simulink model "Automatic_Movement"  (R2015a)
settings: Solver=ode45  StartTime=0.0  StopTime=inf  FixedStep=0.05  RelTol=1e-3
values from neighbouring files (symbols this model uses):
  a_1 = 10.2    [Parameters.m]
  a_2 = 13.1    [Parameters.m]
  a_3 = 5.5    [Parameters.m]
  a_4 = 17    [Parameters.m]
  a_5 = 16.5    [Parameters.m]
  b_1 = 0.243    [Parameters.m]
  b_2 = 0.175    [Parameters.m]
  b_3 = 0.14    [Parameters.m]
  b_4 = 0.14    [Parameters.m]
  b_5 = 0.15    [Parameters.m]
  k1_1 = 2*alpha-a_1    (= 13.8)    [Parameters.m]
  k1_2 = 2*alpha-a_2    (= 10.9)    [Parameters.m]
  k1_3 = 2*alpha-a_3    (= 18.5)    [Parameters.m]
  k1_4 = 2*alpha-a_4    (= 7)    [Parameters.m]
  k1_5 = 2*alpha-a_5    (= 7.5)    [Parameters.m]
  k2_1 = alpha^2-b_1*k1_1    (= 140.6466)    [Parameters.m]
  k2_2 = alpha^2-b_2*k1_2    (= 142.0925)    [Parameters.m]
  k2_3 = alpha^2-b_3*k1_3    (= 141.41)    [Parameters.m]
  k2_4 = alpha^2-b_4*k1_4    (= 143.02)    [Parameters.m]
  k2_5 = alpha^2-b_5*k1_5    (= 142.875)    [Parameters.m]
  Ts = 0.06    [Parameters.m]
  Va = 24    [Parameters.m]
undefined symbols (not defined in the file or in its folder): DiscIntNeverNeededParam, gray, none, strel, videoinput
libraries: simulink x33, arduino_io_lib x28, visiontextngfix x6, visionanalysis x6, visionmorphops x4, visionstatistics x2, visionsinks x2, imaqlib x1
(part 2 of 2)

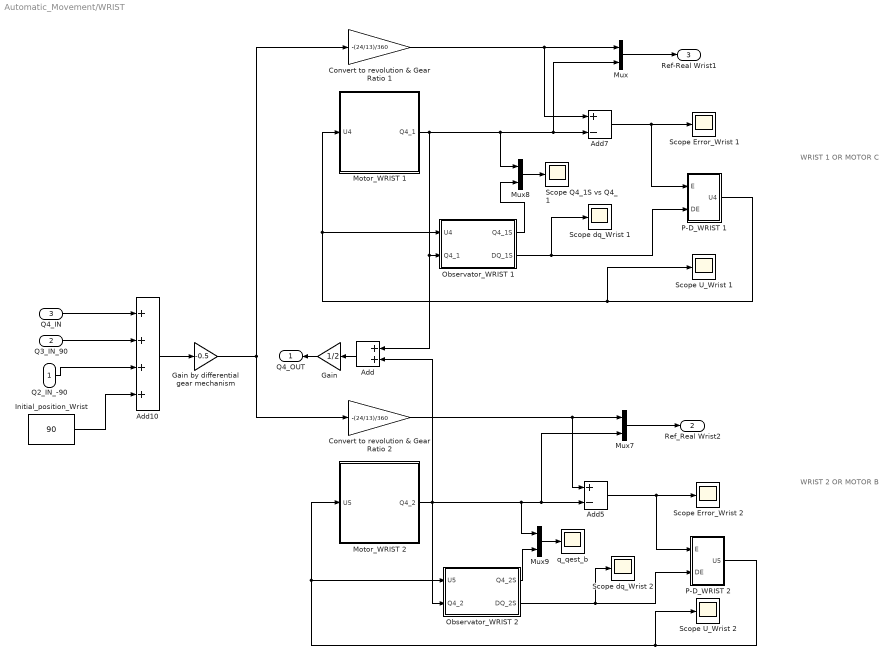
== system Automatic_Movement/WRIST ==
  note: WRIST 1
      | OR
      | MOTOR C
  note: WRIST 2
      | OR
      | MOTOR B
  Q2_IN_-90 : Inport
  "Q3_IN_90 " : Inport  Port=2
  Q4_IN : Inport  Port=3
  Add : Sum
  Add10 : Sum  Inputs=++++
  Add5 : Sum  Inputs=+-
  Add7 : Sum  Inputs=+-
  Convert to revolution & Gear Ratio 1 : Gain  Gain=-(24/13)/360
  Convert to revolution & Gear Ratio 2 : Gain  Gain=-(24/13)/360
  Gain : Gain  Gain=1/2
  Gain by differential gear mechanism : Gain  Gain=-0.5
  Initial_position_Wrist : Constant  Value=90  SampleTime=Ts
  Motor_WRIST 1 : Subsystem
  Motor_WRIST 2 : Subsystem
  Mux{,7..9} (4 alike) : Mux  Inputs=2
  Observator_WRIST 1 : Subsystem
  Observator_WRIST 2 : Subsystem
  P-D_WRIST 1 : Subsystem
  P-D_WRIST 2 : Subsystem
  Scope Error_Wrist 1 : Scope
      settings: TimeRange=auto  MaxDataPoints=5000  SaveName=e_motorc  YMin=-0.01356  YMax=0.08445  SampleTime=-1
  Scope Error_Wrist 2 : Scope
      settings: TimeRange=auto  MaxDataPoints=5000  SaveName=e_motorb  YMin=-0.00284  YMax=0.02557  SampleTime=-1
  Scope Q4_1S vs Q4_1 : Scope
      settings: TimeRange=100  MaxDataPoints=5000  SaveToWorkspace=off  SaveName=ScopeData4  YMin=-0.08445  YMax=0.01356  SampleTime=-1
  Scope U_Wrist 1 : Scope
      settings: TimeRange=auto  MaxDataPoints=5000  SaveName=u_c  YMin=-0.26048  YMax=2.34429  SampleTime=-1
  Scope U_Wrist 2 : Scope
      settings: TimeRange=auto  MaxDataPoints=5000  SaveName=u_b  YMin=-0.19737  YMax=0.74892  SampleTime=-1
  Scope dq_Wrist 1 : Scope
      settings: TimeRange=auto  MaxDataPoints=5000  SaveName=dq_c  YMin=-0.01595  YMax=0.09161  SampleTime=-1
  Scope dq_Wrist 2 : Scope
      settings: TimeRange=auto  MaxDataPoints=5000  SaveName=dq_b  YMin=-0.13693  YMax=0.06105  SampleTime=-1
  q_qest_b : Scope
      settings: TimeRange=100  MaxDataPoints=5000  SaveToWorkspace=off  SaveName=ScopeData5  YMin=-0.00142  YMax=0.01278  SampleTime=-1
  Q4_OUT : Outport
  Ref_Real Wrist2 : Outport  Port=2
  Ref-Real Wrist1 : Outport  Port=3
  wires:
  Observator_WRIST 1/2(DQ_1S) -> Scope dq_Wrist 1/1, P-D_WRIST 1/2(DE)
  P-D_WRIST 1/1(U4) -> Motor_WRIST 1/1(U4), Observator_WRIST 1/1("U4 "), Scope U_Wrist 1/1
  P-D_WRIST 2/1(U5) -> Scope U_Wrist 2/1, Motor_WRIST 2/1(U5), Observator_WRIST 2/1(U5)
  "Q3_IN_90 "/1 -> Add10/2
  Motor_WRIST 1/1(Q4_1) -> Mux/2, Add7/2, Mux8/1, Add/1, Observator_WRIST 1/2(Q4_1)
  Add10/1 -> Gain by differential gear mechanism/1
  Convert to revolution & Gear Ratio 1/1 -> Add7/1, Mux/1
  Add5/1 -> Scope Error_Wrist 2/1, P-D_WRIST 2/1(E)
  Add7/1 -> Scope Error_Wrist 1/1, P-D_WRIST 1/1(E)
  Mux/1 -> Ref-Real Wrist1/1
  Initial_position_Wrist/1 -> Add10/4
  Convert to revolution & Gear Ratio 2/1 -> Mux7/1, Add5/1
  Mux7/1 -> Ref_Real Wrist2/1
  Q4_IN/1 -> Add10/1
  Observator_WRIST 2/1(Q4_2S) -> Mux9/2
  Mux9/1 -> q_qest_b/1
  Observator_WRIST 1/1(Q4_1S) -> Mux8/2
  Motor_WRIST 2/1(Q4_2) -> Add/2, Mux7/2, Add5/2, Mux9/1, Observator_WRIST 2/2(Q4_2)
  Mux8/1 -> Scope Q4_1S vs Q4_1/1
  Gain by differential gear mechanism/1 -> Convert to revolution & Gear Ratio 2/1, Convert to revolution & Gear Ratio 1/1
  Q2_IN_-90/1 -> Add10/3
  Observator_WRIST 2/2(DQ_2S) -> Scope dq_Wrist 2/1, P-D_WRIST 2/2(DE)
  Add/1 -> Gain/1
  Gain/1 -> Q4_OUT/1

== system Automatic_Movement/BODY/Motor_BODY ==
  U1 : Inport
  Arduino Analog Write PWM : arduino_io_lib/Arduino Analog Write  arduinoVar=Temporary arduino variable: Arduino2  arduinoPin=9  T=Ts
  Arduino Digital Write  LEFT : arduino_io_lib/Arduino Digital Write  arduinoVar=Temporary arduino variable: Arduino2  arduinoPin=7  T=Ts
  Arduino Digital Write RIGHT : arduino_io_lib/Arduino Digital Write  arduinoVar=Temporary arduino variable: Arduino2  arduinoPin=6  T=Ts
  Control_Signal : Subsystem
  Encoder Read Body : arduino_io_lib/Encoder Read  arduinoVar=Temporary arduino variable: Arduino2  encNum=2  pinA=21  pinB=20  DbDl=0  T=Ts
  Gear_Ration & Pulses : Gain  Gain=1/(144*24)
  Q1 : Outport
  wires:
  Control_Signal/2(LEFT) -> Arduino Digital Write  LEFT/1
  Gear_Ration & Pulses/1 -> Q1/1
  Control_Signal/1(PWM) -> Arduino Analog Write PWM/1
  Control_Signal/3(RIGHT) -> Arduino Digital Write RIGHT/1
  Encoder Read Body/1 -> Gear_Ration & Pulses/1
  U1/1 -> Control_Signal/1(U1)

== system Automatic_Movement/BODY/Observator_BODY ==
  note: hatx
  note: dot(hatx)
  U1 : Inport
  Q1 : Inport  Port=2
  A : Gain  Gain=[0,1;0,-a_1]  Multiplication=Matrix(K*u)
  Add : Sum  Inputs=+-
  Add1 : Sum  Inputs=+++
  B : Gain  Gain=[0;b_1]  Multiplication=Matrix(K*u)
  C : Gain  Gain=[1,0]  Multiplication=Matrix(K*u)
  Demux : Demux  Outputs=2
  Integrator : Integrator
  K : Gain  Gain=[k1_1;k2_1]  Multiplication=Matrix(K*u)
  Q2_S : Outport
  DQ_S : Outport  Port=2
  wires:
  C/1 -> Add/2
  K/1 -> Add1/3
  B/1 -> Add1/2
  A/1 -> Add1/1
  Add1/1 -> Integrator/1
  Add/1 -> K/1
  Integrator/1 -> Demux/1, C/1, A/1
  Q1/1 -> Add/1
  U1/1 -> B/1
  Demux/1 -> Q2_S/1
  Demux/2 -> DQ_S/1

== system Automatic_Movement/BODY/PI-D_BODY ==
  E : Inport
  DE : Inport  Port=2
  Add : Sum  Inputs=-+
  KD : Gain  Gain=100
  KP : Gain  Gain=400
  Saturation : Saturate  UpperLimit=24  LowerLimit=-24
  U1 : Outport
  wires:
  DE/1 -> KD/1
  KP/1 -> Add/2
  KD/1 -> Add/1
  E/1 -> KP/1
  Add/1 -> Saturation/1
  Saturation/1 -> U1/1

== system Automatic_Movement/ELBOW/Motor_ELBOW ==
  U3 : Inport
  Arduino Analog Write PWM : arduino_io_lib/Arduino Analog Write  arduinoVar=Temporary arduino variable: Arduino2  arduinoPin=11  T=Ts
  Arduino Digital Write Left : arduino_io_lib/Arduino Digital Write  arduinoVar=Temporary arduino variable: Arduino2  arduinoPin=12  T=Ts
  Arduino Digital Write Right : arduino_io_lib/Arduino Digital Write  arduinoVar=Temporary arduino variable: Arduino2  arduinoPin=13  T=Ts
  Control_Signal : Subsystem
  Encoder Read Shoulder : arduino_io_lib/Encoder Read  arduinoVar=Temporary arduino variable: Arduino2  encNum=1  pinA=18  pinB=19  DbDl=0  T=Ts
  Gear_Ration & Pulses : Gain  Gain=1/(144*24)
  Q3 : Outport
  wires:
  Gear_Ration & Pulses/1 -> Q3/1
  Encoder Read Shoulder/1 -> Gear_Ration & Pulses/1
  Control_Signal/1(PWM) -> Arduino Analog Write PWM/1
  Control_Signal/3(RIGHT) -> Arduino Digital Write Right/1
  Control_Signal/2(LEFT) -> Arduino Digital Write Left/1
  U3/1 -> Control_Signal/1(U3)

== system Automatic_Movement/ELBOW/Observator_ELBOW ==
  note: hatx
  note: dot(hatx)
  U3 : Inport
  Q3 : Inport  Port=2
  A : Gain  Gain=[0,1;0,-a_3]  Multiplication=Matrix(K*u)
  Add : Sum  Inputs=+-
  Add1 : Sum  Inputs=+++
  B : Gain  Gain=[0;b_3]  Multiplication=Matrix(K*u)
  C : Gain  Gain=[1,0]  Multiplication=Matrix(K*u)
  Demux : Demux  Outputs=2
  Integrator : Integrator
  K : Gain  Gain=[k1_3;k2_3]  Multiplication=Matrix(K*u)
  Q3_S : Outport
  DQ_S : Outport  Port=2
  wires:
  C/1 -> Add/2
  K/1 -> Add1/3
  B/1 -> Add1/2
  A/1 -> Add1/1
  Add1/1 -> Integrator/1
  Add/1 -> K/1
  Integrator/1 -> A/1, Demux/1, C/1
  Q3/1 -> Add/1
  U3/1 -> B/1
  Demux/1 -> Q3_S/1
  Demux/2 -> DQ_S/1

== system Automatic_Movement/ELBOW/PI-D_ELBOW ==
  E : Inport
  DE : Inport  Port=2
  Add2 : Sum  Inputs=+-
  Add3 : Sum  Inputs=-++
  Add4 : Sum  Inputs=+-
  Discrete-Time Integrator : DiscreteIntegrator  IntegratorMethod=Integration: Trapezoidal  InitialConditionSetting=State (most efficient)  SampleTime=Ts  ICPrevOutput=DiscIntNeverNeededParam  ICPrevScaledInput=DiscIntNeverNeededParam
  KD : Gain  Gain=110
  KI : Gain  Gain=250
  KP : Gain  Gain=385
  Ka : Gain  Gain=700
  Saturation1 : Saturate  UpperLimit=24  LowerLimit=-24
  U3 : Outport
  wires:
  Add3/1 -> Add2/1, Saturation1/1
  DE/1 -> KD/1
  KP/1 -> Add3/2
  KD/1 -> Add3/1
  Add4/1 -> KI/1
  Add2/1 -> Ka/1
  Saturation1/1 -> Add2/2, U3/1
  Ka/1 -> Add4/2
  Discrete-Time Integrator/1 -> Add3/3
  KI/1 -> Discrete-Time Integrator/1
  E/1 -> Add4/1, KP/1

== system Automatic_Movement/SHOULDER /Motor_SHOULDER  ==
  U2 : Inport
  Arduino Analog Write PWM : arduino_io_lib/Arduino Analog Write  arduinoVar=Temporary arduino variable: Arduino2  arduinoPin=10  T=Ts
  Arduino Digital Write Left : arduino_io_lib/Arduino Digital Write  arduinoVar=Temporary arduino variable: Arduino2  arduinoPin=4  T=Ts
  Arduino Digital Write Right : arduino_io_lib/Arduino Digital Write  arduinoVar=Temporary arduino variable: Arduino2  arduinoPin=5  T=Ts
  Control_Signal : Subsystem
  Encoder Read Shoulder : arduino_io_lib/Encoder Read  arduinoVar=Temporary arduino variable: Arduino2  encNum=0  pinA=2  pinB=3  DbDl=0  T=Ts
  Gear_Ration & Pulses : Gain  Gain=1/(144*24)
  Q2 : Outport
  wires:
  Encoder Read Shoulder/1 -> Gear_Ration & Pulses/1
  Gear_Ration & Pulses/1 -> Q2/1
  Control_Signal/3(RIGHT) -> Arduino Digital Write Right/1
  Control_Signal/1(PWM) -> Arduino Analog Write PWM/1
  Control_Signal/2(LEFT) -> Arduino Digital Write Left/1
  U2/1 -> Control_Signal/1(U2)

== system Automatic_Movement/SHOULDER /Observator_SHOULDER ==
  note: hatx
  note: dot(hatx)
  U2 : Inport
  Q2 : Inport  Port=2
  A : Gain  Gain=[0,1;0,-a_2]  Multiplication=Matrix(K*u)
  Add : Sum  Inputs=+-
  Add1 : Sum  Inputs=+++
  B : Gain  Gain=[0;b_2]  Multiplication=Matrix(K*u)
  C : Gain  Gain=[1,0]  Multiplication=Matrix(K*u)
  Demux : Demux  Outputs=2
  Integrator : Integrator
  K : Gain  Gain=[k1_2;k2_2]  Multiplication=Matrix(K*u)
  Q2_S : Outport
  DQ_S : Outport  Port=2
  wires:
  C/1 -> Add/2
  K/1 -> Add1/3
  B/1 -> Add1/2
  A/1 -> Add1/1
  Add1/1 -> Integrator/1
  Add/1 -> K/1
  Integrator/1 -> Demux/1, C/1, A/1
  Q2/1 -> Add/1
  U2/1 -> B/1
  Demux/1 -> Q2_S/1
  Demux/2 -> DQ_S/1

== system Automatic_Movement/SHOULDER /PI-D_SHOULDER ==
  E : Inport
  DE : Inport  Port=2
  Add1 : Sum  Inputs=+-
  Add2 : Sum  Inputs=-++
  Add4 : Sum  Inputs=+-
  Discrete-Time Integrator : DiscreteIntegrator  IntegratorMethod=Integration: Trapezoidal  InitialConditionSetting=State (most efficient)  SampleTime=Ts  ICPrevOutput=DiscIntNeverNeededParam  ICPrevScaledInput=DiscIntNeverNeededParam
  KD : Gain  Gain=126
  KI : Gain  Gain=250
  KP : Gain  Gain=350
  Saturation : Saturate  UpperLimit=24  LowerLimit=-24
  ka : Gain  Gain=700
  U2 : Outport
  wires:
  KP/1 -> Add2/2
  KD/1 -> Add2/1
  DE/1 -> KD/1
  KI/1 -> Discrete-Time Integrator/1
  ka/1 -> Add4/2
  Add1/1 -> ka/1
  Discrete-Time Integrator/1 -> Add2/3
  Add2/1 -> Add1/1, Saturation/1
  Saturation/1 -> U2/1, Add1/2
  Add4/1 -> KI/1
  E/1 -> KP/1, Add4/1

== system Automatic_Movement/Selectors/Selector_phi ==
  OPENING_GRIPPER : Inport
  CLOSING_GRIPPER : Inport  Port=2
  OPEN_SENSOR : Inport  Port=3
  FORCE_SENSOR : Inport  Port=4
  KI_CAMARA_PHI : Inport  Port=5
  KI_FIXED_PHI : Inport  Port=6
  Data Store Read No WorkSpace : DataStoreRead  DataStoreName=No_WorkSpace  SampleTime=Ts
  Logical Operator : Logic  Operator=OR  Inputs=3  AllPortsSameDT=off  OutDataTypeStr=boolean
  Logical Operator1 : Logic  Operator=OR  AllPortsSameDT=off  OutDataTypeStr=boolean
  Logical Operator3 : Logic  Operator=NOT  AllPortsSameDT=off  OutDataTypeStr=boolean
  Logical Operator5 : Logic  Operator=NOT  AllPortsSameDT=off  OutDataTypeStr=boolean
  Logical Operator6 : Logic  AllPortsSameDT=off  OutDataTypeStr=boolean
  Switch1 : Switch  Threshold=1  ZeroCross=off
  Switch8 : Switch  Threshold=1  ZeroCross=off
  K_I_PHI : Outport
  wires:
  KI_CAMARA_PHI/1 -> Switch8/1, Switch1/3
  Logical Operator/1 -> Switch8/2
  Switch8/1 -> K_I_PHI/1
  CLOSING_GRIPPER/1 -> Logical Operator/1
  OPENING_GRIPPER/1 -> Logical Operator1/1
  OPEN_SENSOR/1 -> Logical Operator/2
  KI_FIXED_PHI/1 -> Switch1/1
  Switch1/1 -> Switch8/3
  FORCE_SENSOR/1 -> Logical Operator3/1, Logical Operator1/2
  Logical Operator1/1 -> Switch1/2
  Logical Operator3/1 -> Logical Operator6/2
  Logical Operator5/1 -> Logical Operator6/1
  Data Store Read No WorkSpace/1 -> Logical Operator5/1
  Logical Operator6/1 -> Logical Operator/3

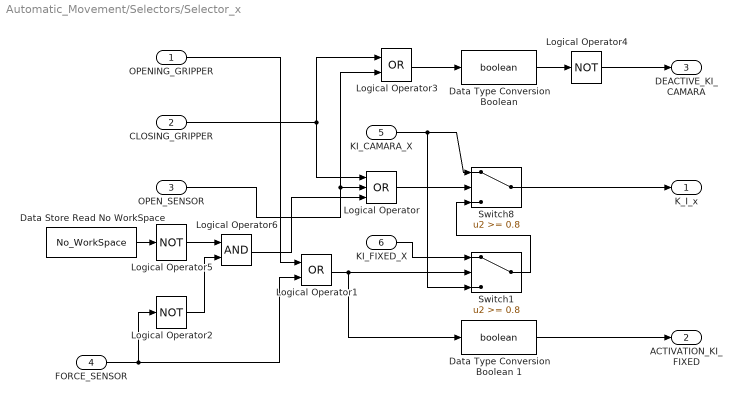
== system Automatic_Movement/Selectors/Selector_x ==
  OPENING_GRIPPER : Inport
  CLOSING_GRIPPER : Inport  Port=2
  OPEN_SENSOR : Inport  Port=3
  FORCE_SENSOR : Inport  Port=4
  KI_CAMARA_X : Inport  Port=5
  KI_FIXED_X : Inport  Port=6
  Data Store Read No WorkSpace : DataStoreRead  DataStoreName=No_WorkSpace  SampleTime=Ts
  Data Type Conversion Boolean 1 : DataTypeConversion  OutDataTypeStr=boolean
  Data Type Conversion Boolean : DataTypeConversion  OutDataTypeStr=boolean
  Logical Operator : Logic  Operator=OR  Inputs=3  AllPortsSameDT=off  OutDataTypeStr=boolean
  Logical Operator1 : Logic  Operator=OR  AllPortsSameDT=off  OutDataTypeStr=boolean
  Logical Operator2 : Logic  Operator=NOT  AllPortsSameDT=off  OutDataTypeStr=boolean
  Logical Operator3 : Logic  Operator=OR  AllPortsSameDT=off  OutDataTypeStr=boolean
  Logical Operator4 : Logic  Operator=NOT  AllPortsSameDT=off  OutDataTypeStr=boolean
  Logical Operator5 : Logic  Operator=NOT  AllPortsSameDT=off  OutDataTypeStr=boolean
  Logical Operator6 : Logic  AllPortsSameDT=off  OutDataTypeStr=boolean
  Switch1 : Switch  Threshold=0.8  ZeroCross=off
  Switch8 : Switch  Threshold=0.8  ZeroCross=off
  K_I_x : Outport
  ACTIVATION_KI_FIXED : Outport  Port=2
  DEACTIVE_KI_CAMARA : Outport  Port=3
  wires:
  KI_CAMARA_X/1 -> Switch8/1, Switch1/3
  Logical Operator/1 -> Switch8/2
  Switch8/1 -> K_I_x/1
  CLOSING_GRIPPER/1 -> Logical Operator3/1, Logical Operator/1
  OPENING_GRIPPER/1 -> Logical Operator1/1
  OPEN_SENSOR/1 -> Logical Operator/2, Logical Operator3/2
  KI_FIXED_X/1 -> Switch1/1
  Switch1/1 -> Switch8/3
  FORCE_SENSOR/1 -> Logical Operator1/2, Logical Operator2/1
  Logical Operator1/1 -> Data Type Conversion Boolean 1/1, Switch1/2
  Data Type Conversion Boolean 1/1 -> ACTIVATION_KI_FIXED/1
  Logical Operator3/1 -> Data Type Conversion Boolean/1
  Data Type Conversion Boolean/1 -> Logical Operator4/1
  Logical Operator4/1 -> DEACTIVE_KI_CAMARA/1
  Data Store Read No WorkSpace/1 -> Logical Operator5/1
  Logical Operator5/1 -> Logical Operator6/1
  Logical Operator2/1 -> Logical Operator6/2
  Logical Operator6/1 -> Logical Operator/3

== system Automatic_Movement/Selectors/Selector_y ==
  "OPENING_GRIPPER " : Inport
  CLOSING_GRIPPER : Inport  Port=2
  OPEN_SENSOR : Inport  Port=3
  FORCE_SENSOR : Inport  Port=4
  CI_CAMARA_y : Inport  Port=5
  KI_FIXED_Y : Inport  Port=6
  Data Store Read No WorkSpace : DataStoreRead  DataStoreName=No_WorkSpace  SampleTime=Ts
  Logical Operator : Logic  Operator=OR  Inputs=3  AllPortsSameDT=off  OutDataTypeStr=boolean
  Logical Operator1 : Logic  Operator=OR  AllPortsSameDT=off  OutDataTypeStr=boolean
  Logical Operator3 : Logic  Operator=NOT  AllPortsSameDT=off  OutDataTypeStr=boolean
  Logical Operator5 : Logic  Operator=NOT  AllPortsSameDT=off  OutDataTypeStr=boolean
  Logical Operator6 : Logic  AllPortsSameDT=off  OutDataTypeStr=boolean
  Switch1 : Switch  Threshold=1  ZeroCross=off
  Switch8 : Switch  Threshold=1  ZeroCross=off
  K_I_Y : Outport
  wires:
  CI_CAMARA_y/1 -> Switch1/3, Switch8/1
  Logical Operator/1 -> Switch8/2
  Switch8/1 -> K_I_Y/1
  CLOSING_GRIPPER/1 -> Logical Operator/1
  "OPENING_GRIPPER "/1 -> Logical Operator1/1
  OPEN_SENSOR/1 -> Logical Operator/2
  KI_FIXED_Y/1 -> Switch1/1
  Switch1/1 -> Switch8/3
  FORCE_SENSOR/1 -> Logical Operator3/1, Logical Operator1/2
  Logical Operator1/1 -> Switch1/2
  Data Store Read No WorkSpace/1 -> Logical Operator5/1
  Logical Operator6/1 -> Logical Operator/3
  Logical Operator3/1 -> Logical Operator6/2
  Logical Operator5/1 -> Logical Operator6/1

== system Automatic_Movement/Selectors/Selector_z ==
  OPENING_GRIPPER : Inport
  CLOSING_GRIPPER : Inport  Port=2
  OPEN_SENSOR : Inport  Port=3
  FORCE_SENSOR : Inport  Port=4
  KI_CAMARA_Z : Inport  Port=5
  KI_FIXED_Z : Inport  Port=6
  Data Store Read No WorkSpace : DataStoreRead  DataStoreName=No_WorkSpace  SampleTime=Ts
  Logical Operator : Logic  Operator=OR  Inputs=3  AllPortsSameDT=off  OutDataTypeStr=boolean
  Logical Operator1 : Logic  Operator=OR  AllPortsSameDT=off  OutDataTypeStr=boolean
  Logical Operator3 : Logic  Operator=NOT  AllPortsSameDT=off  OutDataTypeStr=boolean
  Logical Operator5 : Logic  Operator=NOT  AllPortsSameDT=off  OutDataTypeStr=boolean
  Logical Operator6 : Logic  AllPortsSameDT=off  OutDataTypeStr=boolean
  Switch1 : Switch  Threshold=1  ZeroCross=off
  Switch8 : Switch  Threshold=1  ZeroCross=off
  K_I_Z : Outport
  wires:
  KI_CAMARA_Z/1 -> Switch8/1, Switch1/3
  Logical Operator/1 -> Switch8/2
  Switch8/1 -> K_I_Z/1
  CLOSING_GRIPPER/1 -> Logical Operator/1
  OPENING_GRIPPER/1 -> Logical Operator1/1
  OPEN_SENSOR/1 -> Logical Operator/2
  KI_FIXED_Z/1 -> Switch1/1
  Switch1/1 -> Switch8/3
  FORCE_SENSOR/1 -> Logical Operator1/2, Logical Operator3/1
  Logical Operator1/1 -> Switch1/2
  Logical Operator6/1 -> Logical Operator/3
  Logical Operator3/1 -> Logical Operator6/2
  Logical Operator5/1 -> Logical Operator6/1
  Data Store Read No WorkSpace/1 -> Logical Operator5/1

== system Automatic_Movement/Vision/Enabled and Triggered Subsystem ==
  R_in : Inport
  G_in : Inport  Port=2
  B_in : Inport  Port=3
  Enable : EnablePort
  R_out : Outport
  G_out : Outport  Port=2
  B_out : Outport  Port=3
  wires:
  R_in/1 -> R_out/1
  B_in/1 -> B_out/1
  G_in/1 -> G_out/1

== system Automatic_Movement/Vision/Eval_Circle_R ==
  In1 : Inport
  Compare To Constant : simulink/Logic and Bit Operations/Compare To Constant  relop=>=  const=1.0  OutDataTypeStr=boolean
  Constant : Constant  Value=[1,1]  VectorParams1D=off
  Data Type Conversion1 : DataTypeConversion  OutDataTypeStr=double
  Dot Product : DotProduct  InputSameDT=on  OutDataTypeStr=Inherit: Inherit via internal rule
  Out1 : Outport
  wires:
  Dot Product/1 -> Compare To Constant/1
  Constant/1 -> Dot Product/1
  Data Type Conversion1/1 -> Dot Product/2
  Compare To Constant/1 -> Out1/1
  In1/1 -> Data Type Conversion1/1

== system Automatic_Movement/Vision/Eval_Circle_Y ==
  In1 : Inport
  Compare To Constant : simulink/Logic and Bit Operations/Compare To Constant  relop=>=  const=1.0  OutDataTypeStr=boolean
  Constant : Constant  Value=[1,1]  VectorParams1D=off
  Data Type Conversion1 : DataTypeConversion  OutDataTypeStr=double
  Dot Product : DotProduct  InputSameDT=on  OutDataTypeStr=Inherit: Inherit via internal rule
  Out1 : Outport
  wires:
  Dot Product/1 -> Compare To Constant/1
  Constant/1 -> Dot Product/1
  Data Type Conversion1/1 -> Dot Product/2
  Compare To Constant/1 -> Out1/1
  In1/1 -> Data Type Conversion1/1

== system Automatic_Movement/Vision/Eval_Square_R ==
  In1 : Inport
  Compare To Constant : simulink/Logic and Bit Operations/Compare To Constant  relop=>=  const=1.0  OutDataTypeStr=boolean
  Constant : Constant  Value=[1,1]  VectorParams1D=off
  Data Type Conversion1 : DataTypeConversion  OutDataTypeStr=double
  Dot Product : DotProduct  InputSameDT=on  OutDataTypeStr=Inherit: Inherit via internal rule
  Out1 : Outport
  wires:
  Compare To Constant/1 -> Out1/1
  Constant/1 -> Dot Product/1
  Data Type Conversion1/1 -> Dot Product/2
  Dot Product/1 -> Compare To Constant/1
  In1/1 -> Data Type Conversion1/1

== system Automatic_Movement/Vision/Eval_Square_Y ==
  In1 : Inport
  Compare To Constant : simulink/Logic and Bit Operations/Compare To Constant  relop=>=  const=1.0  OutDataTypeStr=boolean
  Constant : Constant  Value=[1,1]  VectorParams1D=off
  Data Type Conversion1 : DataTypeConversion  OutDataTypeStr=double
  Dot Product : DotProduct  InputSameDT=on  OutDataTypeStr=Inherit: Inherit via internal rule
  Out1 : Outport
  wires:
  Compare To Constant/1 -> Out1/1
  Constant/1 -> Dot Product/1
  Data Type Conversion1/1 -> Dot Product/2
  Dot Product/1 -> Compare To Constant/1
  In1/1 -> Data Type Conversion1/1

== system Automatic_Movement/Vision/Figure_Calculator_R ==
  note: Th_Square
  note: Th_Circle
  "C " : Inport
  Constant1 : Constant  Value=13.6
  Constant4 : Constant  Value=12.5
  Constant5 : Constant  Value=18
  Constant6 : Constant  Value=13.6
  Logical Operator : Logic  AllPortsSameDT=off  OutDataTypeStr=boolean
  Logical Operator2 : Logic  AllPortsSameDT=off  OutDataTypeStr=boolean
  Relational Operator : RelationalOperator  Operator=<=  OutDataTypeStr=boolean
  Relational Operator1 : RelationalOperator  Operator=>  OutDataTypeStr=boolean
  Relational Operator4 : RelationalOperator  Operator=<=  OutDataTypeStr=boolean
  Relational Operator5 : RelationalOperator  Operator=>  OutDataTypeStr=boolean
  Circle : Outport
  Square : Outport  Port=2
  wires:
  Relational Operator/1 -> Logical Operator/1
  Constant4/1 -> Relational Operator/1
  Relational Operator1/1 -> Logical Operator/2
  Logical Operator/1 -> Circle/1
  Constant1/1 -> Relational Operator1/1
  Logical Operator2/1 -> Square/1
  Relational Operator4/1 -> Logical Operator2/1
  Constant5/1 -> Relational Operator5/1
  Relational Operator5/1 -> Logical Operator2/2
  Constant6/1 -> Relational Operator4/1
  "C "/1 -> Relational Operator1/2, Relational Operator/2, Relational Operator4/2, Relational Operator5/2

== system Automatic_Movement/Vision/Figure_Calculator_Y ==
  note: Th_Square
  note: Th_Circle
  "C " : Inport
  Constant1 : Constant  Value=13.6
  Constant4 : Constant  Value=12.5
  Constant5 : Constant  Value=18
  Constant6 : Constant  Value=13.6
  Logical Operator : Logic  AllPortsSameDT=off  OutDataTypeStr=boolean
  Logical Operator2 : Logic  AllPortsSameDT=off  OutDataTypeStr=boolean
  Relational Operator : RelationalOperator  Operator=<=  OutDataTypeStr=boolean
  Relational Operator1 : RelationalOperator  Operator=>  OutDataTypeStr=boolean
  Relational Operator4 : RelationalOperator  Operator=<=  OutDataTypeStr=boolean
  Relational Operator5 : RelationalOperator  Operator=>  OutDataTypeStr=boolean
  Circle : Outport
  Square : Outport  Port=2
  wires:
  Relational Operator/1 -> Logical Operator/1
  Constant4/1 -> Relational Operator/1
  Relational Operator1/1 -> Logical Operator/2
  Logical Operator/1 -> Circle/1
  Constant1/1 -> Relational Operator1/1
  Logical Operator2/1 -> Square/1
  Relational Operator4/1 -> Logical Operator2/1
  Constant5/1 -> Relational Operator5/1
  Relational Operator5/1 -> Logical Operator2/2
  Constant6/1 -> Relational Operator4/1
  "C "/1 -> Relational Operator1/2, Relational Operator/2, Relational Operator4/2, Relational Operator5/2

== system Automatic_Movement/Vision/Filter_R ==
  Bw_in : Inport
  Dilation strel('diamond',2) : visionmorphops/Dilation  nhoodsrc=Specify via dialog  strel=strel('diamond',2)
  Erosion strel('diamond',1) : visionmorphops/Erosion  nhoodsrc=Specify via dialog  strel=strel('diamond',1)
  Bw_out : Outport
  wires:
  Erosion strel('diamond',1)/1 -> Dilation strel('diamond',2)/1
  Bw_in/1 -> Erosion strel('diamond',1)/1
  Dilation strel('diamond',2)/1 -> Bw_out/1

== system Automatic_Movement/Vision/Filter_Y ==
  Bw_in : Inport
  Dilation strel('diamond',2) : visionmorphops/Dilation  nhoodsrc=Specify via dialog  strel=strel('diamond',2)
  Erosion strel('diamond',1) : visionmorphops/Erosion  nhoodsrc=Specify via dialog  strel=strel('diamond',1)
  Bw_out : Outport
  wires:
  Erosion strel('diamond',1)/1 -> Dilation strel('diamond',2)/1
  Bw_in/1 -> Erosion strel('diamond',1)/1
  Dilation strel('diamond',2)/1 -> Bw_out/1

== system Automatic_Movement/Vision/Red_Identi ==
  R : Inport
  G : Inport  Port=2
  B : Inport  Port=3
  Logical Operator : Logic  Inputs=6  AllPortsSameDT=off  OutDataTypeStr=boolean
  Median Filter_Circular_[5 5]_B : visionanalysis/Median Filter  nghbood=[5 5]  outSize=Same as input port I  padType=Circular  padSrc=Specify via dialog  padVal=0  roundingMode=Floor  overflowMode=off
  Median Filter_Circular_[5 5]_G : visionanalysis/Median Filter  nghbood=[5 5]  outSize=Same as input port I  padType=Circular  padSrc=Specify via dialog  padVal=0  roundingMode=Floor  overflowMode=off
  Median Filter_Circular_[5 5]_R : visionanalysis/Median Filter  nghbood=[5 5]  outSize=Same as input port I  padType=Circular  padSrc=Specify via dialog  padVal=0  roundingMode=Floor  overflowMode=off
  Th_max_B : simulink/Logic and Bit Operations/Compare To Constant  relop=<=  const=(150)/255  OutDataTypeStr=boolean
  Th_max_G : simulink/Logic and Bit Operations/Compare To Constant  relop=<=  const=(150)/255  OutDataTypeStr=boolean
  "Th_max_R " : simulink/Logic and Bit Operations/Compare To Constant  relop=<=  const=(225+30)/255  OutDataTypeStr=boolean
  Th_min_B : simulink/Logic and Bit Operations/Compare To Constant  relop=>=  const=(0)/255  OutDataTypeStr=boolean
  Th_min_G : simulink/Logic and Bit Operations/Compare To Constant  relop=>=  const=(0)/255  OutDataTypeStr=boolean
  Th_min_R : simulink/Logic and Bit Operations/Compare To Constant  relop=>=  const=(225-40)/255  OutDataTypeStr=boolean
  BW : Outport
  wires:
  "Th_max_R "/1 -> Logical Operator/2
  Logical Operator/1 -> BW/1
  Th_min_B/1 -> Logical Operator/5
  Th_max_G/1 -> Logical Operator/4
  Th_min_R/1 -> Logical Operator/1
  Th_min_G/1 -> Logical Operator/3
  Th_max_B/1 -> Logical Operator/6
  R/1 -> Median Filter_Circular_[5 5]_R/1
  G/1 -> Median Filter_Circular_[5 5]_G/1
  B/1 -> Median Filter_Circular_[5 5]_B/1
  Median Filter_Circular_[5 5]_R/1 -> "Th_max_R "/1, Th_min_R/1
  Median Filter_Circular_[5 5]_G/1 -> Th_max_G/1, Th_min_G/1
  Median Filter_Circular_[5 5]_B/1 -> Th_max_B/1, Th_min_B/1

== system Automatic_Movement/Vision/Yellow_ide ==
  R : Inport
  G : Inport  Port=2
  B : Inport  Port=3
  Logical Operator : Logic  Inputs=6  AllPortsSameDT=off  OutDataTypeStr=boolean
  Median Filter_Circular_[5 5]_B : visionanalysis/Median Filter  nghbood=[5 5]  outSize=Same as input port I  padType=Circular  padSrc=Specify via dialog  padVal=0  roundingMode=Floor  overflowMode=off
  Median Filter_Circular_[5 5]_G : visionanalysis/Median Filter  nghbood=[5 5]  outSize=Same as input port I  padType=Circular  padSrc=Specify via dialog  padVal=0  roundingMode=Floor  overflowMode=off
  Median Filter_Circular_[5 5]_R : visionanalysis/Median Filter  nghbood=[5 5]  outSize=Same as input port I  padType=Circular  padSrc=Specify via dialog  padVal=0  roundingMode=Floor  overflowMode=off
  Th_max_B : simulink/Logic and Bit Operations/Compare To Constant  relop=<=  const=(200)/255  OutDataTypeStr=boolean
  Th_max_G : simulink/Logic and Bit Operations/Compare To Constant  relop=<=  const=(225+30)/255  OutDataTypeStr=boolean
  Th_max_R : simulink/Logic and Bit Operations/Compare To Constant  relop=<=  const=(225+30)/255  OutDataTypeStr=boolean
  Th_min_B : simulink/Logic and Bit Operations/Compare To Constant  relop=>=  const=(0)/255  OutDataTypeStr=boolean
  "Th_min_G " : simulink/Logic and Bit Operations/Compare To Constant  relop=>=  const=(200)/255  OutDataTypeStr=boolean
  "Th_min_R " : simulink/Logic and Bit Operations/Compare To Constant  relop=>=  const=(200)/255  OutDataTypeStr=boolean
  BW : Outport
  wires:
  Th_max_R/1 -> Logical Operator/2
  Logical Operator/1 -> BW/1
  Th_min_B/1 -> Logical Operator/5
  Th_max_G/1 -> Logical Operator/4
  "Th_min_R "/1 -> Logical Operator/1
  "Th_min_G "/1 -> Logical Operator/3
  Th_max_B/1 -> Logical Operator/6
  G/1 -> Median Filter_Circular_[5 5]_G/1
  R/1 -> Median Filter_Circular_[5 5]_R/1
  B/1 -> Median Filter_Circular_[5 5]_B/1
  Median Filter_Circular_[5 5]_R/1 -> "Th_min_R "/1, Th_max_R/1
  Median Filter_Circular_[5 5]_G/1 -> Th_max_G/1, "Th_min_G "/1
  Median Filter_Circular_[5 5]_B/1 -> Th_max_B/1, Th_min_B/1

== system Automatic_Movement/WRIST/Motor_WRIST 1 ==
  U4 : Inport
  Arduino Analog Write PWM : arduino_io_lib/Arduino Analog Write  arduinoVar=Temporary arduino variable: Arduino1  arduinoPin=10  T=Ts
  Arduino Digital Write Left : arduino_io_lib/Arduino Digital Write  arduinoVar=Temporary arduino variable: Arduino1  arduinoPin=4  T=Ts
  Arduino Digital Write Right : arduino_io_lib/Arduino Digital Write  arduinoVar=Temporary arduino variable: Arduino1  arduinoPin=5  T=Ts
  Control_Signal : Subsystem
  Encoder Read Wrist 1(C) : arduino_io_lib/Encoder Read  arduinoVar=Temporary arduino variable: Arduino1  encNum=1  pinA=19  pinB=18  DbDl=0  T=Ts
  Gear_Ration & Pulses : Gain  Gain=1/(72*48)
  Q4_1 : Outport
  wires:
  Control_Signal/3(RIGHT) -> Arduino Digital Write Right/1
  Control_Signal/1(PWM) -> Arduino Analog Write PWM/1
  Control_Signal/2(LEFT) -> Arduino Digital Write Left/1
  Encoder Read Wrist 1(C)/1 -> Gear_Ration & Pulses/1
  Gear_Ration & Pulses/1 -> Q4_1/1
  U4/1 -> Control_Signal/1(U1)

== system Automatic_Movement/WRIST/Motor_WRIST 2 ==
  U5 : Inport
  Arduino Analog Write PWM : arduino_io_lib/Arduino Analog Write  arduinoVar=Temporary arduino variable: Arduino1  arduinoPin=11  T=Ts
  Arduino Digital Write Left : arduino_io_lib/Arduino Digital Write  arduinoVar=Temporary arduino variable: Arduino1  arduinoPin=13  T=Ts
  Arduino Digital Write Right : arduino_io_lib/Arduino Digital Write  arduinoVar=Temporary arduino variable: Arduino1  arduinoPin=12  T=Ts
  Control_Signal : Subsystem
  Encoder Read Wrist 2 (B) : arduino_io_lib/Encoder Read  arduinoVar=Temporary arduino variable: Arduino1  encNum=0  pinA=3  pinB=2  DbDl=0  T=Ts
  Gear_Ration & Pulses : Gain  Gain=1/(72*22)
  Q4_2 : Outport
  wires:
  Encoder Read Wrist 2 (B)/1 -> Gear_Ration & Pulses/1
  Gear_Ration & Pulses/1 -> Q4_2/1
  Control_Signal/3(RIGHT) -> Arduino Digital Write Right/1
  Control_Signal/1(PWM) -> Arduino Analog Write PWM/1
  Control_Signal/2(LEFT) -> Arduino Digital Write Left/1
  U5/1 -> Control_Signal/1(U1)

== system Automatic_Movement/WRIST/Observator_WRIST 1 ==
  note: hatx
  note: dot(hatx)
  "U4 " : Inport
  Q4_1 : Inport  Port=2
  A : Gain  Gain=[0,1;0,-a_5]  Multiplication=Matrix(K*u)
  Add : Sum  Inputs=+-
  Add1 : Sum  Inputs=+++
  B : Gain  Gain=[0;b_5]  Multiplication=Matrix(K*u)
  C : Gain  Gain=[1,0]  Multiplication=Matrix(K*u)
  Demux : Demux  Outputs=2
  Integrator : Integrator
  K : Gain  Gain=[k1_5;k2_5]  Multiplication=Matrix(K*u)
  Q4_1S : Outport
  DQ_1S : Outport  Port=2
  wires:
  C/1 -> Add/2
  K/1 -> Add1/3
  B/1 -> Add1/2
  A/1 -> Add1/1
  Add1/1 -> Integrator/1
  Add/1 -> K/1
  Integrator/1 -> Demux/1, C/1, A/1
  Q4_1/1 -> Add/1
  "U4 "/1 -> B/1
  Demux/1 -> Q4_1S/1
  Demux/2 -> DQ_1S/1

== system Automatic_Movement/WRIST/Observator_WRIST 2 ==
  note: hatx
  note: dot(hatx)
  U5 : Inport
  Q4_2 : Inport  Port=2
  A : Gain  Gain=[0,1;0,-a_4]  Multiplication=Matrix(K*u)
  Add : Sum  Inputs=+-
  Add1 : Sum  Inputs=+++
  B : Gain  Gain=[0;b_4]  Multiplication=Matrix(K*u)
  C : Gain  Gain=[1,0]  Multiplication=Matrix(K*u)
  Demux : Demux  Outputs=2
  Integrator : Integrator
  K : Gain  Gain=[k1_4;k2_4]  Multiplication=Matrix(K*u)
  Q4_2S : Outport
  DQ_2S : Outport  Port=2
  wires:
  C/1 -> Add/2
  K/1 -> Add1/3
  B/1 -> Add1/2
  A/1 -> Add1/1
  Add1/1 -> Integrator/1
  Add/1 -> K/1
  Integrator/1 -> Demux/1, C/1, A/1
  Q4_2/1 -> Add/1
  U5/1 -> B/1
  Demux/1 -> Q4_2S/1
  Demux/2 -> DQ_2S/1

== system Automatic_Movement/WRIST/P-D_WRIST 1 ==
  E : Inport
  DE : Inport  Port=2
  Add11 : Sum  Inputs=-+
  "KD " : Gain  Gain=80
  KP : Gain  Gain=300
  Saturation : Saturate  UpperLimit=24  LowerLimit=-24
  U4 : Outport
  wires:
  E/1 -> KP/1
  "KD "/1 -> Add11/1
  DE/1 -> "KD "/1
  Add11/1 -> Saturation/1
  KP/1 -> Add11/2
  Saturation/1 -> U4/1

== system Automatic_Movement/WRIST/P-D_WRIST 2 ==
  E : Inport
  DE : Inport  Port=2
  Add12 : Sum  Inputs=-+
  KD : Gain  Gain=150
  KP : Gain  Gain=400
  Saturation : Saturate  UpperLimit=24  LowerLimit=-24
  U5 : Outport
  wires:
  E/1 -> KP/1
  KD/1 -> Add12/1
  KP/1 -> Add12/2
  Add12/1 -> Saturation/1
  DE/1 -> KD/1
  Saturation/1 -> U5/1

== system Automatic_Movement/BODY/Motor_BODY/Control_Signal ==
  note: pwm a la entreda enable
  U1 : Inport
  Abs : Abs
  Constant : Constant
  Constant1 : Constant  Value=0
  Constant2 : Constant
  Constant3 : Constant  Value=0
  Gain : Gain  Gain=-1
  Scope : Scope
      settings: TimeRange=auto  MaxDataPoints=5000  SaveToWorkspace=off  SaveName=ScopeData  YMin=-10  YMax=10  SampleTime=-1  DataFormat=Array
  Sign : Signum
  Switch : Switch  Threshold=0.9  ZeroCross=off
  Switch1 : Switch  Threshold=0.9  ZeroCross=off
  Voltage to bits : Gain  Gain=255/Va
  PWM : Outport
  LEFT : Outport  Port=2
  RIGHT : Outport  Port=3
  wires:
  Switch/1 -> LEFT/1
  Gain/1 -> Switch1/2
  Voltage to bits/1 -> Sign/1, Abs/1, Scope/1
  Constant/1 -> Switch/1
  Constant1/1 -> Switch/3
  Switch1/1 -> RIGHT/1
  Abs/1 -> PWM/1
  U1/1 -> Voltage to bits/1
  Sign/1 -> Switch/2, Gain/1
  Constant2/1 -> Switch1/1
  Constant3/1 -> Switch1/3

== system Automatic_Movement/ELBOW/Motor_ELBOW/Control_Signal ==
  U3 : Inport
  Abs : Abs
  Constant : Constant
  Constant1 : Constant  Value=0
  Constant2 : Constant
  Constant3 : Constant  Value=0
  Gain : Gain  Gain=-1
  Sign : Signum
  Switch : Switch  Threshold=0.9  ZeroCross=off
  Switch1 : Switch  Threshold=0.9  ZeroCross=off
  Voltage to bits : Gain  Gain=255/Va
  PWM : Outport
  LEFT : Outport  Port=2
  RIGHT : Outport  Port=3
  wires:
  Switch/1 -> LEFT/1
  Gain/1 -> Switch1/2
  Voltage to bits/1 -> Sign/1, Abs/1
  Constant/1 -> Switch/1
  Constant1/1 -> Switch/3
  Switch1/1 -> RIGHT/1
  Abs/1 -> PWM/1
  U3/1 -> Voltage to bits/1
  Sign/1 -> Switch/2, Gain/1
  Constant2/1 -> Switch1/1
  Constant3/1 -> Switch1/3

== system Automatic_Movement/SHOULDER /Motor_SHOULDER /Control_Signal ==
  note: pwm a la entreda enable
  U2 : Inport
  Abs : Abs
  Constant : Constant
  Constant1 : Constant  Value=0
  Constant2 : Constant
  Constant3 : Constant  Value=0
  Gain : Gain  Gain=-1
  Sign : Signum
  Switch : Switch  Threshold=0.9  ZeroCross=off
  Switch1 : Switch  Threshold=0.9  ZeroCross=off
  Voltage to bits : Gain  Gain=255/Va
  PWM : Outport
  LEFT : Outport  Port=2
  RIGHT : Outport  Port=3
  wires:
  Switch/1 -> LEFT/1
  Gain/1 -> Switch1/2
  Voltage to bits/1 -> Sign/1, Abs/1
  Constant/1 -> Switch/1
  Constant1/1 -> Switch/3
  Switch1/1 -> RIGHT/1
  Abs/1 -> PWM/1
  U2/1 -> Voltage to bits/1
  Sign/1 -> Switch/2, Gain/1
  Constant2/1 -> Switch1/1
  Constant3/1 -> Switch1/3

== system Automatic_Movement/WRIST/Motor_WRIST 1/Control_Signal ==
  U1 : Inport
  Abs : Abs
  Constant : Constant
  Constant1 : Constant  Value=0
  Constant2 : Constant
  Constant3 : Constant  Value=0
  Gain : Gain  Gain=-1
  Scope : Scope
      settings: TimeRange=auto  MaxDataPoints=5000  SaveToWorkspace=off  SaveName=ScopeData  YMin=-10  YMax=10  SampleTime=-1  DataFormat=Array
  Sign : Signum
  Switch : Switch  Threshold=0.9  ZeroCross=off
  Switch1 : Switch  Threshold=0.9  ZeroCross=off
  Voltage to bits : Gain  Gain=255/Va
  PWM : Outport
  LEFT : Outport  Port=2
  RIGHT : Outport  Port=3
  wires:
  Switch/1 -> LEFT/1
  Gain/1 -> Switch1/2
  Voltage to bits/1 -> Sign/1, Abs/1, Scope/1
  Constant/1 -> Switch/1
  Constant1/1 -> Switch/3
  Switch1/1 -> RIGHT/1
  Abs/1 -> PWM/1
  U1/1 -> Voltage to bits/1
  Sign/1 -> Switch/2, Gain/1
  Constant2/1 -> Switch1/1
  Constant3/1 -> Switch1/3

== system Automatic_Movement/WRIST/Motor_WRIST 2/Control_Signal ==
  U1 : Inport
  Abs : Abs
  Constant : Constant
  Constant1 : Constant  Value=0
  Constant2 : Constant
  Constant3 : Constant  Value=0
  Gain : Gain  Gain=-1
  Scope : Scope
      settings: TimeRange=auto  MaxDataPoints=5000  SaveToWorkspace=off  SaveName=ScopeData  YMin=-10  YMax=10  SampleTime=-1  DataFormat=Array
  Sign : Signum
  Switch : Switch  Threshold=0.9  ZeroCross=off
  Switch1 : Switch  Threshold=0.9  ZeroCross=off
  Voltage to bits : Gain  Gain=255/Va
  PWM : Outport
  LEFT : Outport  Port=2
  RIGHT : Outport  Port=3
  wires:
  Switch/1 -> LEFT/1
  Gain/1 -> Switch1/2
  Voltage to bits/1 -> Sign/1, Abs/1, Scope/1
  Constant/1 -> Switch/1
  Constant1/1 -> Switch/3
  Switch1/1 -> RIGHT/1
  Abs/1 -> PWM/1
  U1/1 -> Voltage to bits/1
  Sign/1 -> Switch/2, Gain/1
  Constant2/1 -> Switch1/1
  Constant3/1 -> Switch1/3

== matlab function Automatic_Movement/Forward/MATLAB Function ==
  data: q1 input; x output; q2 input; q3 input; q4 input; y output; z output; phi output
function [x,y,z,phi] = fcn(q1,q2,q3,q4)

d1=37;
a1=22;
a2=22;
a3=14;

x=cosd(q1)*[a1*cosd(q2)+a2*cosd(q2+q3)+a3*cosd(q2+q3+q4)];
y=sind(q1)*[a1*cosd(q2)+a2*cosd(q2+q3)+a3*cosd(q2+q3+q4)];
z=d1+a1*sind(q2)+a2*sind(q2+q3)+a3*sind(q2+q3+q4);
phi=q2+q3+q4;

== matlab function Automatic_Movement/MATLAB Function  ==
  data: x input; q1 output; y input; z input; phi input; q2 output; q3 output; q4 output
function [q1,q2,q3,q4] = fcn(x,y,z,phi)

%Lengths of the links.
d1=37;
a1=22;
a2=22;
a3=14;

% Inverse kinematics
s=z-d1;
r=sqrt(x^2+y^2); 
tr = (phi*(pi/180));
pwx = r-(a3*cos(tr));
pwy = s-(a3*sin(tr));
D = (pwx^2 + pwy^2 -a1^2 - a2^2 ) / (2*a1*a2);

% Angular coordinates	
q1=atan2d(y,x);
q3 = atan2d(-sqrt(1-D^2),D);
t3r = (q3*pi/180);
q2 = atan2d(pwy,pwx) - atan2d(a2*sin(t3r),a1+a2*cos(t3r));
q4=phi-q2-q3;

== matlab function Automatic_Movement/Vision/MATLAB Function1 ==
  data: center input; variable output
function variable = transpuesta(center)
%High camara
h_camara=700;
%High object
h_objeto=55;
%Split Matrix
c1=center(:,1); %%x
c2=center(:,2); %%y
%Distance center WorkSpace
d=[200;200];
d1=typecast(d,'double');
%Correction x position 
c12=-c1+d1;
x_error=(h_objeto/h_camara)*c12;
x_objeto=c12-x_error;
%Correction y position
%Split vector
c21=c2(1,:);
c22=c2(2,:);
y_error1=(h_objeto/h_camara)*c21*(1/2);
y_error2=(h_objeto/h_camara)*c22*(1/2);
%Condition of correction object_1
if(c21>70)
  y_objeto1=c21-y_error1;
else
  y_objeto1=c21+y_error1;   
end
%Condition of correction object_2
if(c22>70)
  y_objeto2=c22-y_error2;
else
  y_objeto2=c22+y_error2;   
end
y_objeto=[y_objeto1;y_objeto2];
%Ouput x_object  and y_object
n=[x_objeto,y_objeto];
%Transpose
v=n';
variable = [v];

== matlab function Automatic_Movement/Vision/MATLAB Function2 ==
  data: center input; variable output
function variable = transpuesta(center)
%High camara
h_camara=700;
%High object
h_objeto=55;
%Split Matrix
c1=center(:,1); %%x
c2=center(:,2); %%y
%Distance center WorkSpace
d=[200;200];
d1=typecast(d,'double');
%Correction x position 
c12=-c1+d1;
x_error=(h_objeto/h_camara)*c12;
x_objeto=c12-x_error;
%Correction y position
%Split vector
c21=c2(1,:);
c22=c2(2,:);
y_error1=(h_objeto/h_camara)*c21*(1/2);
y_error2=(h_objeto/h_camara)*c22*(1/2);
%Condition of correction object_1
if(c21>70)
  y_objeto1=c21-y_error1;
else
  y_objeto1=c21+y_error1;   
end
%Condition of correction object_2
if(c22>70)
  y_objeto2=c22-y_error2;
else
  y_objeto2=c22+y_error2;   
end
y_objeto=[y_objeto1;y_objeto2];
%Ouput x_object  and y_object
n=[x_objeto,y_objeto];
%Transpose
v=n';
variable = [v];

== matlab function Automatic_Movement/Vision/MATLAB Function3 ==
  data: center input; location output
function location = transpuesta(center)
%Split Matrix
c1=center(:,1); %%x
c2=center(:,2);  %%y

dx=[25;25];
dy=35;
%Convert dx and dy to double
dx1=typecast(dx,'double');
dy1=typecast(dy,'double');
%Correction x
x=c1-dx1;
%Correction y
c2_1=c2(1,:);
c2_2=c2(2,:);

if (c2_1>=70)
    c2_11=c2_1-dy1;
else 
    c2_11=c2_1+dy1;
end

if (c2_2>=70)
    c2_21=c2_2-dy1;
else 
    c2_21=c2_2+dy1;
end
y=[c2_11;c2_21];
%Ouput x_object  and y_object
n=[x,y];
location = [n];

== matlab function Automatic_Movement/C_O_G/MATLAB Function2 ==
  data: u1 input; y1 output; u2 input; y2 output
function [y1,y2]= fcn(u1,u2)
%#codegen
y1 = 0;
y2 = 0;
if (u1==1)
    y1 = 1;
    y2 = 0;  
elseif(u2==1)
    y1 = 0;
    y2 = 1;
else
    y1 = 0;
    y2 = 0;
end
end

== matlab function Automatic_Movement/Vision/MATLAB Function4 ==
  data: center input; location output
function location = transpuesta(center)
%Split Matrix
c1=center(:,1); %%x
c2=center(:,2);  %%y

dx=[25;25];
dy=35;
%Convert dx and dy to double
dx1=typecast(dx,'double');
dy1=typecast(dy,'double');
%Correction x
x=c1-dx1;
%Correction y
c2_1=c2(1,:);
c2_2=c2(2,:);

if (c2_1>=70)
    c2_11=c2_1-dy1;
else 
    c2_11=c2_1+dy1;
end

if (c2_2>=70)
    c2_21=c2_2-dy1;
else 
    c2_21=c2_2+dy1;
end
y=[c2_11;c2_21];
%Ouput x_object  and y_object
n=[x,y];
location = [n];
